simulink model "Segway_Regelung_Roboter"  (R2016b)
settings: Solver=VariableStepAuto  StartTime=0.0  StopTime=3  RelTol=1e-3  EnableMultiTasking=on
values from neighbouring files (symbols this model uses):
  F_Roboter = [0      -m2*l_SP*r_Rad ... (first row only)    [Robotersimulation_Teil_6.m]
  R_Kipp_Roboter = R_kipp    [Robotersimulation_Teil_6.m]
undefined symbols (not defined in the file or in its folder): C_Roboter, G_mot, M_Roboter, sigbuilder_block, v_Regler_Roboter
libraries: simulink x1
settings Model: Creator=Nitzsche  LastModifiedBy=Stephan
settings DataIOCC: LimitDataPoints=on
settings OptimizationCC: LifeSpan=inf
settings DebuggingCC: AllowSymbolicDim=off  SFUnexpectedBacktrackingDiag=warning  SFNoUnconditionalDefaultTransitionDiag=warning  SFExecutionAtInitializationDiag=none
settings ModelReferenceCC: PropagateSignalLabelsOutOfModel=off
settings GRTTargetCC: TargetLangStandard=C89/C90 (ANSI)
settings ConfigComp: CovMetricSettings=dw  CovHtmlReporting=on  CovSaveCumulativeToWorkspaceVar=on  CovSaveSingleToWorkspaceVar=on  CovExternalEMLEnable=off

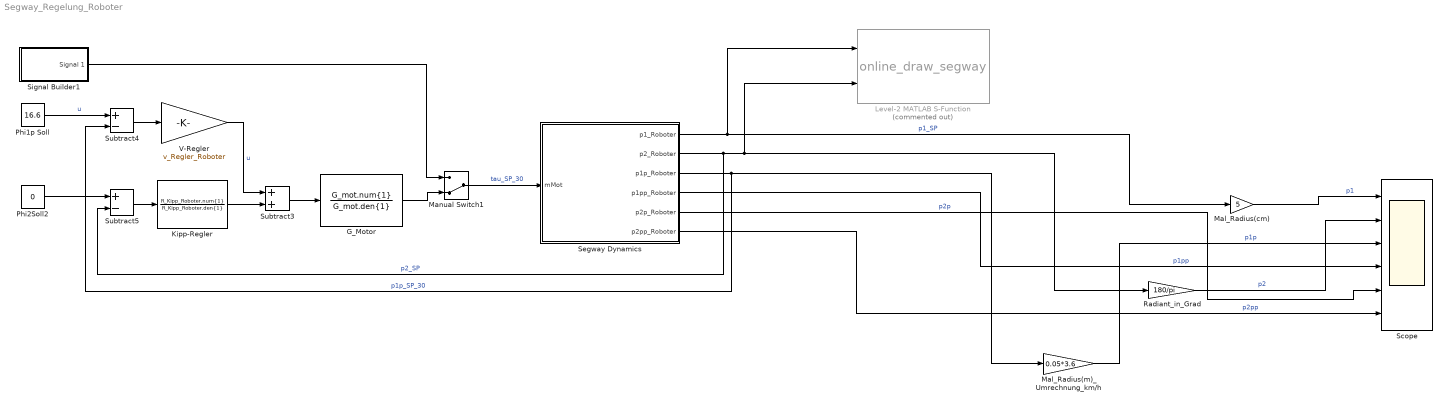
== system Segway_Regelung_Roboter ==
  G_Motor : TransferFcn  Numerator=G_mot.num{1}  Denominator=G_mot.den{1}
  Kipp-Regler : TransferFcn  Numerator=R_Kipp_Roboter.num{1}  Denominator=R_Kipp_Roboter.den{1}
  Level-2 MATLAB S-Function : M-S-Function  Commented=on  FunctionName=online_draw_segway
  "Mal_Radius(cm) " : Gain  Gain=5
  Mal_Radius(m)_Umrechnung_km/h : Gain  Gain=0.05*3.6
  Manual Switch1 : ManualSwitch  CurrentSetting=0
  Phi1p Soll : Constant  Value=16.6
  Phi2Soll2 : Constant  Value=0
  Radiant_in_Grad : Gain  Gain=180/pi
  Scope : Scope  NumInputPorts=6
  Segway Dynamics : Subsystem
  Signal Builder1 : Subsystem  Tag=STV Subsys  LoadFcn=sigbuilder_block('load');  StartFcn=sigbuilder_block('start');  StopFcn=sigbuilder_block('stop');  ClipboardFcn=sigbuilder_block('clipboard');  mask(Sigbuilder block){tuvar=[0:10]}
      mask help: Simulink:masks:SigbuilderBlock_MD
      mask init:
      | if ~strcmp(get_param(bdroot(gcbh),'SimulationStatus'),'stopped') tuvar = sigbuilder_block('maskInit'); end
      settings: CopyFcn=sigbuilder_block('copy');  DeleteFcn=sigbuilder_block('delete');  ModelCloseFcn=sigbuilder_block('modelClose');  PreSaveFcn=sigbuilder_block('preSave');  PauseFcn=sigbuilder_block('pause');  ContinueFcn=sigbuilder_block('continue');  NameChangeFcn=sigbuilder_block('namechange');  OpenFcn=sigbuilder_block('open',[191.25 133.5 827.25 303.75 ]);  CloseFcn=sigbuilder_block('close');
      mask Display: plot(0, 0, 100, 100,[2, 2, 32, 32, 2], [68, 8, 8, 68, 68],[32, 2], [38, 38], [32, 19, 2],[53, 60, 44], [32, 17, 17, 2],[16, 16, 31, 31]);txt = getActiveGroup(gcbh);text(2, 100, txt,'verticalAlignment', 'top');
  Subtract3 : Sum
  Subtract4 : Sum  Inputs=+-
  Subtract5 : Sum  Inputs=+-
  V-Regler : Gain  Gain=v_Regler_Roboter
  wires:
  Phi1p Soll/1 -> Subtract4/1  "u"
  G_Motor/1 -> Manual Switch1/2
  V-Regler/1 -> Subtract3/1  "u"
  Subtract3/1 -> G_Motor/1
  Kipp-Regler/1 -> Subtract3/2
  Subtract5/1 -> Kipp-Regler/1
  Manual Switch1/1 -> Segway Dynamics/1(mMot)  "tau_SP_30"
  Subtract4/1 -> V-Regler/1
  Segway Dynamics/1(p1_Roboter) -> Level-2 MATLAB S-Function/1, "Mal_Radius(cm) "/1  "p1_SP"
  Segway Dynamics/3(p1p_Roboter) -> Subtract4/2, Mal_Radius(m)_Umrechnung_km/h/1  "p1p_SP_30"
  Segway Dynamics/4(p1pp_Roboter) -> Scope/4  "p1pp"
  Segway Dynamics/2(p2_Roboter) -> Subtract5/2, Level-2 MATLAB S-Function/2, Radiant_in_Grad/1  "p2_SP"
  Segway Dynamics/5(p2p_Roboter) -> Scope/5  "p2p"
  Segway Dynamics/6(p2pp_Roboter) -> Scope/6  "p2pp"
  Signal Builder1/1(Signal 1) -> Manual Switch1/1
  Phi2Soll2/1 -> Subtract5/1
  "Mal_Radius(cm) "/1 -> Scope/1  "p1"
  Radiant_in_Grad/1 -> Scope/2  "p2"
  Mal_Radius(m)_Umrechnung_km/h/1 -> Scope/3  "p1p"

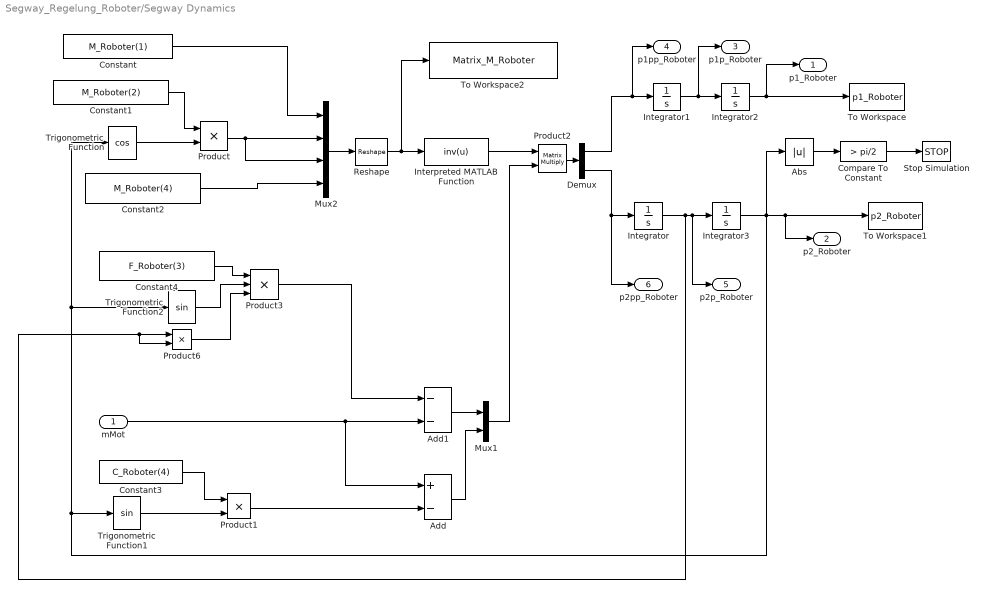
== system Segway_Regelung_Roboter/Segway Dynamics ==
  mMot : Inport
  Abs : Abs
  Add : Sum  Inputs=+-
  Add1 : Sum  Inputs=--
  Compare To Constant : simulink/Logic and Bit Operations/Compare To Constant  relop=>  const=pi/2  OutDataTypeStr=boolean
  Constant : Constant  Value=M_Roboter(1)
  Constant1 : Constant  Value=M_Roboter(2)
  Constant2 : Constant  Value=M_Roboter(4)
  Constant3 : Constant  Value=C_Roboter(4)
  Constant4 : Constant  Value=F_Roboter(3)
  Demux : Demux  Outputs=2
  Integrator{,1..3} (4 alike) : Integrator
  Interpreted MATLAB Function : MATLABFcn  MATLABFcn=inv(u)  Output1D=off
  Mux1 : Mux  Inputs=2
  Mux2 : Mux
  Product : Product
  Product1 : Product
  Product2 : Product  Multiplication=Matrix(*)
  Product3 : Product  Inputs=3
  Product6 : Product
  Reshape : Reshape  OutputDimensionality=Customize  OutputDimensions=[2,2]
  Stop Simulation : Stop
  To Workspace : ToWorkspace  VariableName=p1_Roboter  SaveFormat=Timeseries  SampleTime=0.01
  To Workspace1 : ToWorkspace  VariableName=p2_Roboter  SaveFormat=Timeseries  SampleTime=0.01
  To Workspace2 : ToWorkspace  VariableName=Matrix_M_Roboter  SampleTime=-1
  Trigonometric Function : Trigonometry  Operator=cos
  Trigonometric Function1 : Trigonometry
  Trigonometric Function2 : Trigonometry
  p1_Roboter : Outport
  p2_Roboter : Outport  Port=2
  p1p_Roboter : Outport  Port=3
  p1pp_Roboter : Outport  Port=4
  p2p_Roboter : Outport  Port=5
  p2pp_Roboter : Outport  Port=6
  wires:
  Constant/1 -> Mux2/1
  Product1/1 -> Add/2
  Constant1/1 -> Product/1
  Add/1 -> Mux1/2
  Constant2/1 -> Mux2/4
  Integrator1/1 -> p1p_Roboter/1, Integrator2/1
  Integrator/1 -> p2p_Roboter/1, Integrator3/1, Product6/2, Product6/1
  Abs/1 -> Compare To Constant/1
  Integrator3/1 -> Trigonometric Function2/1, Trigonometric Function/1, Trigonometric Function1/1, p2_Roboter/1, To Workspace1/1, Abs/1
  Trigonometric Function1/1 -> Product1/2
  Product/1 -> Mux2/3, Mux2/2
  Trigonometric Function/1 -> Product/2
  Constant3/1 -> Product1/1
  Demux/1 -> p1pp_Roboter/1, Integrator1/1
  mMot/1 -> Add1/2, Add/1
  Integrator2/1 -> To Workspace/1, p1_Roboter/1
  Reshape/1 -> To Workspace2/1, Interpreted MATLAB Function/1
  Compare To Constant/1 -> Stop Simulation/1
  Mux2/1 -> Reshape/1
  Mux1/1 -> Product2/2
  Interpreted MATLAB Function/1 -> Product2/1
  Product2/1 -> Demux/1
  Demux/2 -> p2pp_Roboter/1, Integrator/1
  Constant4/1 -> Product3/1
  Trigonometric Function2/1 -> Product3/2
  Product6/1 -> Product3/3
  Add1/1 -> Mux1/1
  Product3/1 -> Add1/1

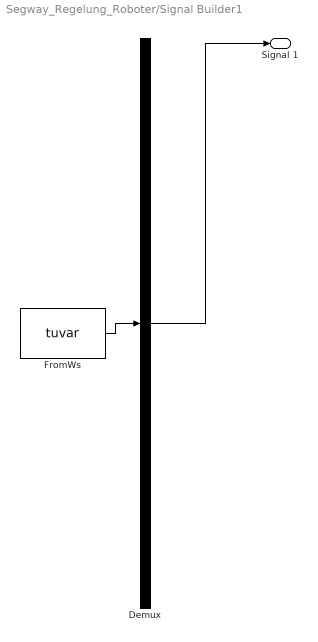
== system Segway_Regelung_Roboter/Signal Builder1 ==
  Demux : Demux  Tag=STV Demux  Outputs=1
  FromWs : FromWorkspace  Tag=STV FromWs  VariableName=tuvar  SampleTime=0
      SigBuilderData=|
      | common.afterFinalStr = 'Extrapolate'
      | common.sampleTime = 0
      | dataSet.timeRange = [0 2]
      | dataSet.name = 'Group 1'
      | sbobj.Groups.Name = 'Group 1'
      | sbobj.Groups.Signals.Name = 'Signal 1'
      | sbobj.Groups.Signals.XData = [0 0.23 0.23 0.395 0.395 0.43 0.43 1.795 1.795 2]
      | sbobj.Groups.Signals.YData = [0 0 0.011 0.011 0 0 -0.095 -0.095 0 0]
      | sbobj.Groups.TimeRange = [0 2]
  Signal 1 : Outport  Tag=STV Outport
  wires:
  Demux/1 -> Signal 1/1
  FromWs/1 -> Demux/1
